simulink model "jtcMonitor"  (Simulink 8.0)
settings: Solver=FixedStepDiscrete  StartTime=0.0  StopTime=inf  RelTol=1e-3
libraries: WBCLibrary x1
settings Model: Creator=icub  LastModifiedBy=icub

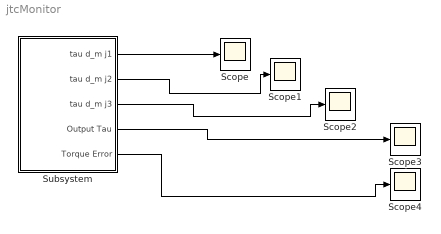
== system jtcMonitor ==
  Scope{,1..4} (5 alike) : Scope
      Scope2 settings: SaveName=ScopeData2
      Scope3 settings: SaveName=ScopeData3
      Scope4 settings: SaveName=ScopeData4
  Subsystem : Subsystem  mask{moduleName='jtc'}
      mask prompts: moduleName "module name"
  wires:
  Subsystem/1(tau d_m j1) -> Scope/1
  Subsystem/2(tau d_m j2) -> Scope1/1
  Subsystem/3(tau d_m j3) -> Scope2/1
  Subsystem/4(Output Tau) -> Scope3/1
  Subsystem/5(Torque Error) -> Scope4/1

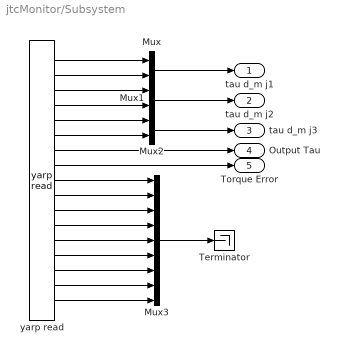
== system jtcMonitor/Subsystem ==
  Mux : Mux  Inputs=2
  Mux1 : Mux  Inputs=2
  Mux2 : Mux  Inputs=2
  Mux3 : Mux  Inputs=9
  Terminator : Terminator
  yarp read : WBCLibrary/Utilities/yarp read  from=['/' moduleName '/monitor:o']  to='...'  num=17
  tau d_m j1 : Outport
  tau d_m j2 : Outport  Port=2
  tau d_m j3 : Outport  Port=3
  Output Tau : Outport  Port=4
  Torque Error : Outport  Port=5
  wires:
  yarp read/9 -> Mux3/1
  yarp read/7 -> Output Tau/1
  yarp read/6 -> Mux2/2
  yarp read/3 -> Mux1/1
  yarp read/17 -> Mux3/9
  yarp read/16 -> Mux3/8
  yarp read/1 -> Mux/1
  yarp read/14 -> Mux3/6
  yarp read/4 -> Mux1/2
  yarp read/11 -> Mux3/3
  yarp read/2 -> Mux/2
  yarp read/15 -> Mux3/7
  yarp read/13 -> Mux3/5
  yarp read/5 -> Mux2/1
  yarp read/10 -> Mux3/2
  Mux1/1 -> tau d_m j2/1
  Mux/1 -> tau d_m j1/1
  yarp read/12 -> Mux3/4
  Mux2/1 -> tau d_m j3/1
  yarp read/8 -> Torque Error/1
  Mux3/1 -> Terminator/1
